simulink model "battery_charger"  (R2020a)
settings: Solver=VariableStepAuto  StartTime=0.0  StopTime=10.0  RelTol=1e-3
undefined symbols (not defined in the file): Ion, Lithium
libraries: powerlib x8, electricdrivelib x1, simulink x1, powerlib_meascontrol x1
settings Model: Creator=Reaga  LastModifiedBy=Reaga
settings DebuggingCC: UnconnectedInputMsg=none  UnconnectedOutputMsg=none  UnconnectedLineMsg=none
settings ModelReferenceCC: EnableRefExpFcnMdlSchedulingChecks=off
settings RTWCC: Description=Generic Real-Time Target
settings ConfigComp: CovBoundaryAbsTol=1.0e-5

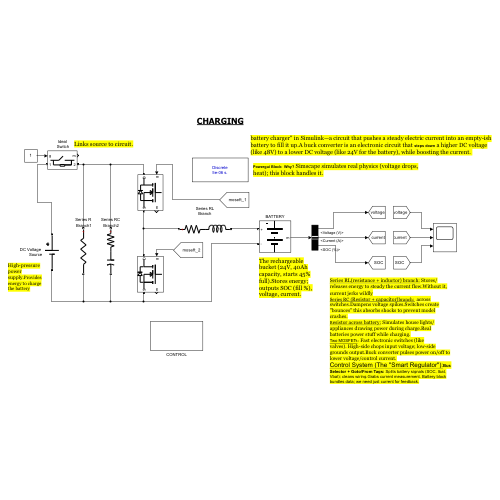
[thumbnail: Simulink's stored preview of the top-level diagram]
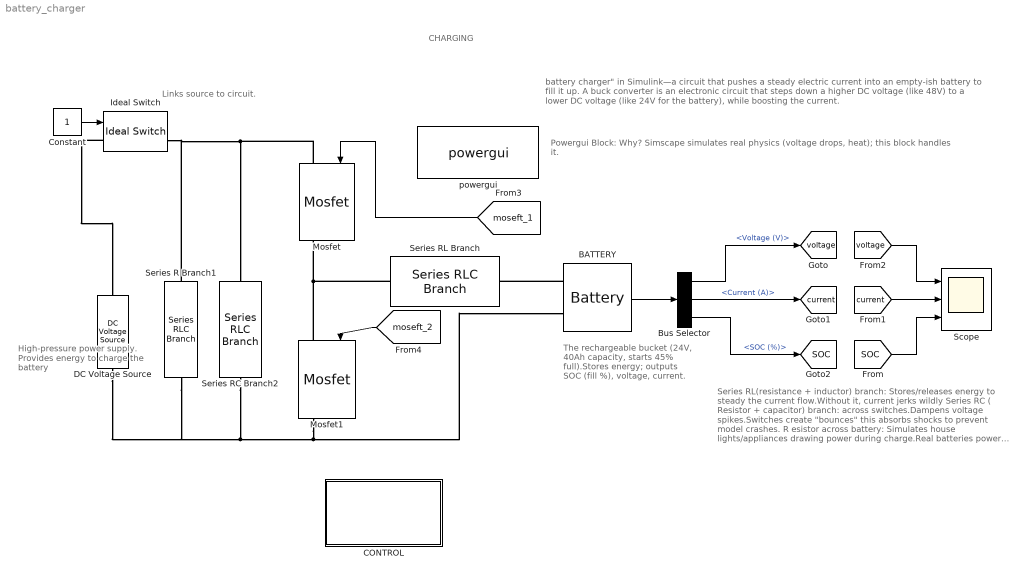
== system battery_charger ==
  note: Links source to circuit.
  note: Series RL(resistance + inductor) branch: Stores/releases energy to steady the current flow.Without it, current jerks wildly
      | Series RC ( Resistor + capacitor) branch: across switches.Dampens voltage spikes.Switches create "bounces" this absorbs shocks to prevent model crashes.
      | R esistor across battery: Simulates house lights/appliances drawing power during charge.Real batteries power stuff while charging.
      | Two MOSFETs : Fast electronic switches (like valves). High-side chops input voltage; low-side grounds output.Buck converter pulses power on/off to lower voltage/control current.
      | C ontrol System (The "Smart Regulator"): Bus Selector + Goto/From Tags: Splits battery signals (SOC, Ibat, Vbat); cleans wiring.Grabs current measurement. Battery block bundles data; we need just current for feedback.
  note: The rechargeable bucket (24V, 40Ah capacity, starts 45% full).Stores energy; outputs SOC (fill %), voltage, current.
  note: High-pressure power supply. Provides energy to charge the battery
  note: Powergui Block: Why? Simscape simulates real physics (voltage drops, heat); this block handles it.
  note: battery charger" in Simulink—a circuit that pushes a steady electric current into an empty-ish battery to fill it up. A buck converter is an electronic circuit that steps down a higher DC voltage (like 48V) to a lower DC voltage (like 24V for the battery), while boosting the current.
  note: CHARGING
  " BATTERY" : electricdrivelib/Extra Sources/Battery  BatType=Lithium-Ion  NomV=24  NomQ=40  SOC=45  Batt_Tr=1  PresetModel=on  MaxQ=40  MinV=18  FullV=27.9357  Dis_rate=17.3913  R=0.006  Normal_OP=36.1739  expZone="[25.9293      1.96522]"
  Bus Selector : BusSelector  OutputSignals=Voltage (V),Current (A),SOC (%)
  CONTROL : Subsystem
  Constant : Constant
  DC Voltage Source : powerlib/Electrical Sources/DC Voltage Source  Amplitude=48  Measurements=None
  Ideal Switch : powerlib/Power Electronics/Ideal Switch  Ron=0.001  Lon=0  IC=0  Rs=1e5  Cs=inf  Measurements=on
  Mosfet : powerlib/Power Electronics/Mosfet  Ron=0.1  Lon=0  Rd=0.01  Vfd=0  IC=0  Rs=1e5  Cs=inf  Measurements=on
  Mosfet1 : powerlib/Power Electronics/Mosfet  Ron=0.1  Lon=0  Rd=0.01  Vfd=0  IC=0  Rs=1e5  Cs=inf  Measurements=on
  Scope : Scope  NumInputPorts=3
  Series R Branch1 : powerlib/Elements/Series RLC Branch  LConnTagsString=__new0  RConnTagsString=__new0  BranchType=R  Resistance=5  Inductance=5.76e-4  SetiL0=off  InitialCurrent=0  Capacitance=1e-6  Setx0=off  InitialVoltage=0  Measurements=None
  Series RC Branch2 : powerlib/Elements/Series RLC Branch  LConnTagsString=__new0  RConnTagsString=__new0  BranchType=RC  Resistance=0.01  Inductance=5.76e-4  SetiL0=off  InitialCurrent=0  Capacitance=1000e-6  Setx0=off  InitialVoltage=0  Measurements=None
  Series RL Branch : powerlib/Elements/Series RLC Branch  LConnTagsString=__new0  RConnTagsString=__new0  BranchType=RL  Resistance=0.05  Inductance=5.76e-4  SetiL0=off  InitialCurrent=0  Capacitance=1e-6  Setx0=off  InitialVoltage=0  Measurements=None
  powergui : powerlib/powergui  Priority=1  SimulationMode=Discrete  SampleTime=5e-6  frequency=60  Iterations=50  frequencyindice=0  Pbase=100e6  ErrMax=1e-4  UnitsV=kV  UnitsW=MW  buscounter=0  FunctionMessages=off  echomessages=off  EnableUseOfTLC=off  CurrentSourceSwitches=off  DisableSnubberDevices=off  DisableRonSwitches=off  DisableVfSwitches=off  DisplayEquations=off  AutomaticDiscreteSolvers=off  SolverType=Tustin/Backward Euler (TBE)  Interpol=off  ExternalGateDelay=off  methode=off  Ts=100  x0status=blocks  SPID=on  SwTol=0  HookPort=off  NonlinearTolerance=1e-4  nMaxIteration=100  ContinueOnMaxIteration=off  RestoreLinks=warning  ResistiveCurrentMeasurement=off  Frange=[0:2:500]  Ylog=off  Xlog=on  ShowGrid=off  save=off  variable=ZData  structure=0  ZoomFFT=off  StartTime=0.0  cycles=1  DisplayStyle=1  fundamental=60  FreqAxis=off  MaxFrequency=1000  frequencyindicesteady=1  RmsSteady=1  display=off
  tag scope: SOC=global, current=global, voltage=global
  wires:
  Constant/1 -> Ideal Switch/1
  " BATTERY"/1 -> Bus Selector/1
  Bus Selector/1 -> [voltage]  "<Voltage (V)>"
  Bus Selector/2 -> [current]  "<Current (A)>"
  Bus Selector/3 -> [SOC]  "<SOC (%)>"
  [moseft_1] -> Mosfet/1
  [moseft_2] -> Mosfet1/1
  [voltage] -> Scope/1
  [current] -> Scope/2
  [SOC] -> Scope/3
  connections:
  " BATTERY"/LConn1 -- Series RL Branch/RConn1
  Mosfet1/LConn1 -- Series RL Branch/LConn1 -- Mosfet/RConn1
  Mosfet1/RConn1 -- DC Voltage Source/LConn1 -- Series R Branch1/RConn1 -- Series RC Branch2/RConn1 -- " BATTERY"/LConn2
  Mosfet/LConn1 -- Series R Branch1/LConn1 -- Ideal Switch/RConn1 -- Series RC Branch2/LConn1
  Ideal Switch/LConn1 -- DC Voltage Source/RConn1

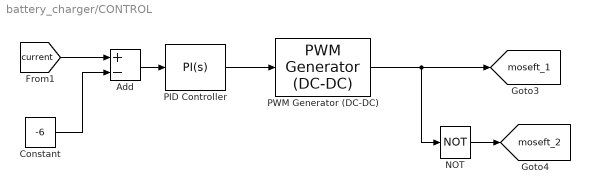
== system battery_charger/CONTROL ==
  Add : Sum  Inputs=+-
  Constant : Constant  Value=-6
  NOT : Logic  Operator=NOT  IconShape=distinctive  AllPortsSameDT=off  OutDataTypeStr=boolean
  PID Controller : simulink/Continuous/PID Controller  Controller=PI  Form=Parallel  TimeDomain=Continuous-time  UseExternalTs=off  SampleTime=-1  IntegratorMethod=Forward Euler  FilterMethod=Forward Euler  ControllerParametersSource=internal  P=0.005  I=10  D=0  N=100  UseFilter=on  TunerSelectOption=Transfer Function Based (PID Tuner App)  InitialConditionSource=internal  InitialConditionForIntegrator=0.54  InitialConditionForFilter=0  DifferentiatorICPrevScaledInput=0  ExternalReset=none  TrackingMode=off  Kt=1  LimitOutput=on  UpperSaturationLimit=0.975  LowerSaturationLimit=0  LinearizeAsGain=on  AntiWindupMode=none  Kb=1  POutMin=[]  POutMax=[]  IOutMin=[]  IOutMax=[]  DOutMin=[]  DOutMax=[]  NOutMin=[]  NOutMax=[]  SumOutMin=[]  SumOutMax=[]  SaturationOutMin=[]  SaturationOutMax=[]  PParamMin=[]  PParamMax=[]  IParamMin=[]  IParamMax=[]  DParamMin=[]  DParamMax=[]  NParamMin=[]  NParamMax=[]  KbParamMin=[]  KbParamMax=[]  KtParamMin=[]  KtParamMax=[]  KbOutMin=[]  KbOutMax=[]  KtOutMin=[]  KtOutMax=[]  IntegratorOutMin=[]  IntegratorOutMax=[]  FilterOutMin=[]  FilterOutMax=[]  SumI1OutMin=[]  SumI1OutMax=[]  SumI2OutMin=[]  SumI2OutMax=[]  SumI3OutMin=[]  SumI3OutMax=[]  SumI4OutMin=[]  SumI4OutMax=[]  SumDOutMin=[]  SumDOutMax=[]  DifferentiatorOutMin=[]  DifferentiatorOutMax=[]  FilterDiffOutCoefMin=[]  FilterDiffOutCoefMax=[]  ReciprocalOutMin=[]  ReciprocalOutMax=[]  SumDenOutMin=[]  SumDenOutMax=[]  SumNumOutMin=[]  SumNumOutMax=[]  DivideOutMin=[]  DivideOutMax=[]  UdiffTsProdOutMin=[]  UdiffTsProdOutMax=[]  NTsProdOutMin=[]  NTsProdOutMax=[]  UintegralTsProdOutMin=[]  UintegralTsProdOutMax=[]  UngainTsProdOutMin=[]  UngainTsProdOutMax=[]  IntegratorContinuousStateAttributes=''  IntegratorStateMustResolveToSignalObject=off  IntegratorRTWStateStorageClass=Auto  FilterContinuousStateAttributes=''  FilterStateMustResolveToSignalObject=off  FilterRTWStateStorageClass=Auto  ParallelPVariant=InternalParameters  IdealPVariant=Disabled  IVariant=InternalParameters  DVariant=Disabled  IntegratorVariant=Continuous  SatVariant=Enabled  AWVariant=Passthrough  PCopyVariant=Disabled  TRVariant=Disabled  FdbkBlocksVariant=Forward  IdealPFdbkVariant=Disabled  SatFdbkVariant=Disabled  DerivativeFilterVariant=Disabled  NVariant=Disabled  NCopyVariant=Disabled_SignalSpec  FilterICVariant=Disabled  IntegratorICVariant=InternalICs  ExternalResetVariant=Disabled  TRSumVariant=Passthrough  SumFdbkVariant=Disabled  SumVariant=Sum_PI  TsampFilterVariant=InternalTs  TsampNgainVariant=Passthrough  TsampIntegralVariant=Disabled_SignalSpec
  PWM Generator (DC-DC) : powerlib_meascontrol/Pulse & Signal Generators/PWM Generator (DC-DC)  Fsw=10e3  Ts=5e-6
  tag scope: moseft_1=global, moseft_2=global
  wires:
  PWM Generator (DC-DC)/1 -> NOT/1, [moseft_1]
  PID Controller/1 -> PWM Generator (DC-DC)/1
  Add/1 -> PID Controller/1
  NOT/1 -> [moseft_2]
  Constant/1 -> Add/2
  [current] -> Add/1
